simulink model "kart"  (R2025b)
settings: Solver=VariableStepAuto  StartTime=0.0  StopTime=10.0  RelTol=1e-3
libraries: slrealtimeutilitieslib x1, instrumentseriallib x1
settings Model: Creator=Lenovo  LastModifiedBy=Lenovo

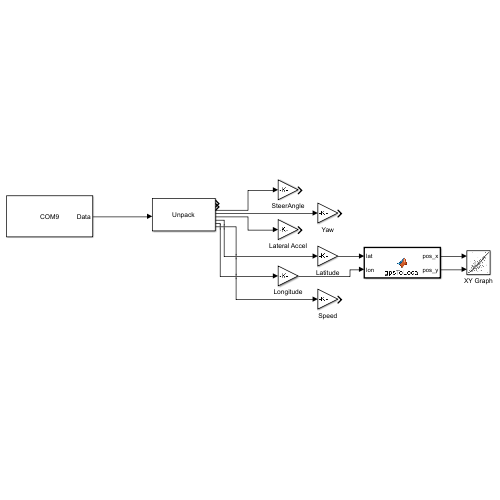
[thumbnail: Simulink's stored preview of the top-level diagram]
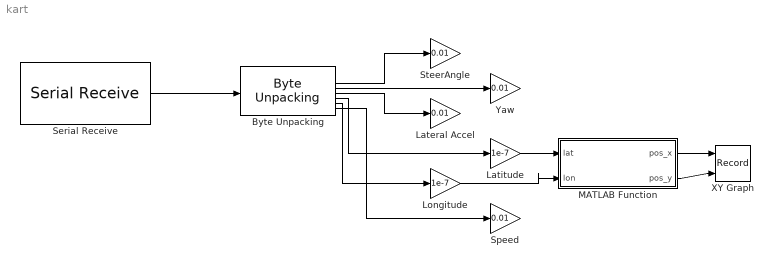
== system kart ==
  Byte Unpacking : slrealtimeutilitieslib/Byte Unpacking  MaskUnpackedDataTypes={'uint32', 'int16', 'int16', 'int16', 'int16', 'int32', 'int32', 'uint16'}  MaskUnpackedDataSizes={[1], [1], [1], [1], [1], [1], [1], [1]}  MaskAlignment=1
  Lateral Accel : Gain  Gain=0.01
  Latitude : Gain  Gain=1e-7
  Longitude : Gain  Gain=1e-7
  MATLAB Function : MATLAB Function  TreatAsAtomicUnit=on
  Serial Receive : instrumentseriallib/Serial Receive  Priority=1  PortSel=COM9  Port=COM9  ComPort=COM9  DataType=uint8  SaveDataType=uint8  ToggleHeader=on  Header=[170]  ToggleDataSize=on  DataSize=[22 1]  ToggleTerminator=off  Terminator=<none>  CustomTerminator=[]  InputFormat=Column major  EnableBlockingMode=on  ActionDataUnavailable=Output last received value  ActionWhenDataUnavailable=Output last received value  CustomValue=0  SampleTime=0.02  SimulateUsing=Interpreted execution  BlockInModel=on  aMode=1  LibraryInUse=instrumentlib
  Speed : Gain  Gain=0.01
  SteerAngle : Gain  Gain=0.01
  XY Graph : Record  NumPorts=2.0  FileSettingsInternal="{\"entries\":[{\"content\":{\"excelSettings\":{\"content\":{},\"type\":\"Streamout.ExcelSettings\"},\"parquetSettings\":{\"content\":{},\"type\":\"Streamout.ParquetSettings\"}},\"type\":\"Streamout.FileSettingStorage\",\"uuid\":\"\"}],\"packageUris\":[\"http:\\/\\/schema.mathworks.com\\/mf0\\/streamout_blocks\\/R2020a\"],\"version\":\"1.0\"}"  FrameSettings=[0, 0]  Layout=[1 1]  SignalsInternal="{\"entries\":[{\"content\":{\"signals\":[{\"content\":{\"blockPath\":[],\"dimensions\":[1],\"domain\":\"\",\"lineColor\":\"#a2142f\",\"plots\":[ 1 ],\"port\":1,\"signalID\":1,\"signalName\":\"XY Graph:1\"},\"type\":\"RecordBlkView.Signal\",\"uuid\":\"\"},{\"content\":{\"blockPath\":[],\"dimensions\":[1],\"domain\":\"\",\"lineColor\":\"#139fff\",\"plots\":[ 1 ],\"port\":2,\"signalID\":2,\"signalName\":\"XY Graph:2\"},\"type\":\"RecordBlkView.Signal\",\"uuid\":\"\"}]},\"type\":\"RecordBlkView.InputSignals\",\"uuid\":\"\"}],\"packageUris\":[\"http:\\/\\/schema.mathworks.com\\/mf0\\/streamout_blocks\\/R2020a\"],\"version\":\"1.0\"}"  VisualizationBindings="{\"xyplotplugin\":{\"info\":[{\"series\":[{\"bindingParametersList\":[{\"parameter\":\"X-Axis\",\"signalID\":1,\"signalName\":\"XY Graph:1\"},{\"parameter\":\"Y-Axis\",\"signalID\":2,\"signalName\":\"XY Graph:2\"}],\"seriesID\":0}],\"subplotID\":1}]}}"  CompatibilityTag=XY
  Yaw : Gain  Gain=0.01
  wires:
  Serial Receive/1 -> Byte Unpacking/1
  Byte Unpacking/3 -> SteerAngle/1
  Byte Unpacking/4 -> Yaw/1
  Byte Unpacking/5 -> Lateral Accel/1
  Byte Unpacking/6 -> Latitude/1
  Byte Unpacking/7 -> Longitude/1
  Byte Unpacking/8 -> Speed/1
  Latitude/1 -> MATLAB Function/1(lat)
  Longitude/1 -> MATLAB Function/2(lon)
  MATLAB Function/1(pos_x) -> XY Graph/1
  MATLAB Function/2(pos_y) -> XY Graph/2

== matlab function kart/MATLAB Function ==
  data: lat input; pos_x output; lon input; pos_y output
function [pos_x, pos_y] = gpsToLocal(lat, lon)
    % Reference Point (Alwar/Home Base)
    % These should match the lat0/lon0 in your Python script
    lat0 = 30.0000000; 
    lon0 = 76.0000000;
    
    % Conversion Factors
    % 1 degree of latitude is approx 111,111 meters
    pos_y = (lat - lat0) * 111111;
    
    % Longitude distance shrinks as you move away from the equator
    pos_x = (lon - lon0) * (111111 * cosd(lat0));
end
